simulink model "Rotacceleration"  (R2018a)
settings: Solver=VariableStepAuto  StartTime=0.0  StopTime=10.0  RelTol=1e-3
settings Model: Creator=shubham mishra  LastModifiedBy=shubham mishra

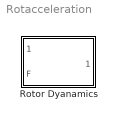
== system Rotacceleration ==
  " Rotor Dyanamics" : MATLAB Function  TreatAsAtomicUnit=on

== matlab function Rotacceleration/ Rotor Dyanamics ==
  data: Torque input; RotAccelearation output; F input
function RotAccelearation = fcn(Torque, F)
Moment = [0 0 0];
RotAcceleration=[0 0 0];
I=[0.003,0.003,0.007];
Moment(1)=(F(3)+F(4))*0.237/2-(F(1)+F(2))*0.237/2;
Moment(2)=(F(3)+F(2))*0.237/2-(F(1)+F(4))*0.237/2;
Moment(3)=Torque(4)-Torque(1)+Torque(2)-Torque(3);
for i=1:3
    RotAccelearation(i)
end
